simulink model "untitled"  (R2018b)
settings: Solver=VariableStepAuto  StartTime=0.0  StopTime=10.0  RelTol=1e-3
libraries: simulink x1
settings Model: Creator=Princess  LastModifiedBy=Princess

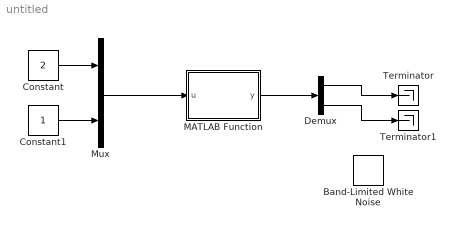
== system untitled ==
  Band-Limited White Noise : simulink/Sources/Band-Limited White Noise  Cov=[0.1]  Ts=0.1  seed=[23341]
  Constant : Constant  Value=2
  Constant1 : Constant
  Demux : Demux  Outputs=2
  MATLAB Function : MATLAB Function  TreatAsAtomicUnit=on
  Mux : Mux  Inputs=2
  Terminator : Terminator
  Terminator1 : Terminator
  wires:
  Constant1/1 -> Mux/2
  Constant/1 -> Mux/1
  Mux/1 -> MATLAB Function/1(u)
  MATLAB Function/1(y) -> Demux/1
  Demux/1 -> Terminator/1
  Demux/2 -> Terminator1/1

== matlab function untitled/MATLAB Function ==
  data: u input; y output
function y = fcn(u)
if u(1) > u(2)
    y = [1,2];
else
    y=[22,11];
end
